simulink model "43_BusNetworkElectricityTransmissionModel"  (R2023b)
settings: Solver=VariableStepAuto  StartTime=0.0  StopTime=0.8  RelTol=1e-3
model workspace (MAT data in the model file):
  BESS_Fp_KDroop = 0.025
  BESS_KSI = 817
  BESS_PWM_fs = 560
  BESS_P_Ki = 0.5
  BESS_P_Kp = 0.0636
  BESS_Pnom = 3000000
  BESS_Q_Ki = 1
  BESS_Q_Kp = 0.0257
  BESS_Vd_Ki = 850
  BESS_Vd_Kp = 0.216
  BESS_Vnom = 1000
  BESS_Vq_KDroop = 0.025
  BESS_Vq_Ki = 850
  BESS_Vq_Kp = 0.216
  Compensation_Ki = 30
  Compensation_Kp = 3
  DC_Ki = 400
  DC_Kp = 8
  F = 0.01
  Flux_min = 0.5
  Grid_Freq_PWM = 2700
  Grid_Ireg_Ki = 5
  Grid_Ireg_Kp = 0.83
  Grid_Ireg_lim = 1.1
  Grid_Modindex_Upper = 1.1
  Grid_conv_Imax = 0.8
  H = 0.685
  Idref_max = 0.9
  Iqref_Tc = 0.3
  Ki_Var = 0.05
  Ki_Vreg = 20
  Ksh = 1.1
  L_pu = 0.3
  Llr = 0.16
  Lls = 0.18
  Lm = 2.9
  LowLoad_P = 130
  Nb_wt = 6
  P_mech = 1080000
  PeakShav_P = 200
  Pitch_Ki = 0
  Pitch_Kp = 150
  Pitch_Max = 27
  Pitch_Tc = 0.01
  Pitch_rate = 10
  Q_Filt = 50
  R_pu = 0.003
  Rotor_Freq_PWM = 1620
  Rotor_Ireg_Ki = 8
  Rotor_Ireg_Kp = 0.6
  Rotor_Ireg_lim = 0.1
  Rotor_Modindex_Upper = 2
  Rr = 0.016
  Rs = 0.023
  SOCBESS : Simulink.Parameter (value not decoded)
  T_set = 0.0001
  Tp = 5e-05
  Ts = 5e-06
  Var_C_Filt = 720000
  Var_reg_max = 1.1
  Var_reg_min = 0.9
  WT_Coeff = [0.645 116 0.4 5 21 0.00912 0.08 0.035]
  WT_H = 4.32
  WT_IGBTRon = 5.931
  WT_Param = [91.204 10143]
  Wind_Freq_Filt = 10000
  Wind_Freq_nom = 60
  Wind_P_nom = 1200000
  Wind_Rotor_V_nom = 1950
  Wind_V_nom = 500
  Zeta_Filt = 0.707106781187
  init = [-0.2 0 0 0 0 0 0 0]
  p = 3
  torque0 = 0.83
  v_Ki = 0.1
  v_Kp = 3.6
  v_Max = 1.2
  v_Min = 0.7
  v_T = 5
  vreg_max = 1
  wind_VDC_nom = 1150
  wt0 = 1.2
undefined symbols (not defined in the file): D1, D11, Delta, DiscIntNeverNeededParam, Iabc, Ion, Lithium, P, Q, Vabc
libraries: powerlib_extras x156, spsSeriesRLCBranchLib x66, spsLoadFlowBusLib x43, spsThreePhaseSeriesRLCLoadLib x33, spsThreePhaseTransformerTwoWindingsLib x32, spsThreePhaseVIMeasurementLib x30, simulink_extras x30, spsDistributedParametersLineLib x22, spsGenericPowerSystemStabilizerLib x20, spsSynchronousMachinepuStandardLib x10, spsExcitationSystemLib x10, spsHydraulicTurbineandGovernorLib x10
(part 6 of 19)

== system 43_BusNetworkElectricityTransmissionModel/ 41.4 MW Wind Generation/41.4 MW Wind Farm ==
  10.35 MW Wind Turbine 1 : Subsystem
  10.35 MW Wind Turbine 2 : Subsystem
  10.35 MW Wind Turbine 3 : Subsystem
  10.35 MW Wind Turbine 4 : Subsystem
  11.5 MVA 20KV :500V Transformer {1..4} (4 alike) : spsThreePhaseTransformerTwoWindingsLib/Three-Phase Transformer (Two Windings)  Winding1Connection=Delta (D1)  Winding2Connection=Yn  CoreType=Three single-phase transformers  SetSaturation=off  Hysteresis=off  DataFile='hysteresis'  SetInitialFlux=off  Measurements=None  UNITS=pu  NominalPower=[ 1.15e7 , 60 ]  Winding1=[ 20e3 , 0.002 , 0.08 ]  Winding2=[ 500 , 0.002 , 0.08 ]  Rm=500  Lm=500  L0=0.5  Saturation=[ 0,0 ; 0.0024,1.2 ; 1.0,1.52 ]  InitialFluxes=[ 0.8 , -0.8 , 0.7 ]  BreakLoop=off  DiscreteSolver=Trapezoidal iterative  DataType=off  TransfoNumber=1
  Control System : Subsystem
  Ground{,1..3} (4 alike) : spsGroundLib/Ground  LConnTagsString=a
  Load Flow Bus1 : spsLoadFlowBusLib/Load Flow Bus  LConnTagsString=a  Phases=single  Connectors=on one side  ID=BUS_31  Vbase=20e3  Vref=1  Vangle=0  VLF=1  VLFb=1  VLFc=1  angleLF=0  angleLFb=0  angleLFc=0
  Load Flow Bus2 : spsLoadFlowBusLib/Load Flow Bus  LConnTagsString=a  Phases=single  Connectors=on one side  ID=BUS_32  Vbase=20e3  Vref=1  Vangle=0  VLF=1  VLFb=1  VLFc=1  angleLF=0  angleLFb=0  angleLFc=0
  Load Flow Bus3 : spsLoadFlowBusLib/Load Flow Bus  LConnTagsString=a  Phases=single  Connectors=on one side  ID=BUS_33  Vbase=20e3  Vref=1  Vangle=0  VLF=1  VLFb=1  VLFc=1  angleLF=0  angleLFb=0  angleLFc=0
  Load Flow Bus4 : spsLoadFlowBusLib/Load Flow Bus  LConnTagsString=a  Phases=single  Connectors=on one side  ID=BUS_34  Vbase=500  Vref=1  Vangle=0  VLF=1  VLFb=1  VLFc=1  angleLF=0  angleLFb=0  angleLFc=0
  Load Flow Bus5 : spsLoadFlowBusLib/Load Flow Bus  LConnTagsString=a  Phases=single  Connectors=on one side  ID=BUS_35  Vbase=500  Vref=1  Vangle=0  VLF=1  VLFb=1  VLFc=1  angleLF=0  angleLFb=0  angleLFc=0
  Load Flow Bus6 : spsLoadFlowBusLib/Load Flow Bus  LConnTagsString=a  Phases=single  Connectors=on one side  ID=BUS_30  Vbase=20e3  Vref=1  Vangle=0  VLF=1  VLFb=1  VLFc=1  angleLF=0  angleLFb=0  angleLFc=0
  Load Flow Bus7 : spsLoadFlowBusLib/Load Flow Bus  LConnTagsString=a  Phases=single  Connectors=on one side  ID=BUS_36  Vbase=500  Vref=1  Vangle=0  VLF=1  VLFb=1  VLFc=1  angleLF=0  angleLFb=0  angleLFc=0
  Load Flow Bus8 : spsLoadFlowBusLib/Load Flow Bus  LConnTagsString=a  Phases=single  Connectors=on one side  ID=BUS_37  Vbase=500  Vref=1  Vangle=0  VLF=1  VLFb=1  VLFc=1  angleLF=0  angleLFb=0  angleLFc=0
  Series RLC Branch{,1..3} (4 alike) : spsSeriesRLCBranchLib/Series RLC Branch  LConnTagsString=__new0  RConnTagsString=__new0  BranchType=R  Resistance=66  Inductance=0  SetiL0=off  InitialCurrent=0  Capacitance=0  Setx0=off  InitialVoltage=0  Measurements=None
  Three-Phase PI Section Line{,1..3} (4 alike) : spsThreePhasePISectionLineLib/Three-Phase PI Section Line  LConnTagsString=a|b|c  RConnTagsString=A|B|C  Length=0.5  Frequency=60  Resistances=[ 0.01273 0.3864]  Inductances="[ 0.9337e-3  4.1264e-3]"  Capacitances=[12.74e-9 7.751e-9]
  Three-Phase Series RLC Load{,1..3} (4 alike) : spsThreePhaseSeriesRLCLoadLib/Three-Phase Series RLC Load  LConnTagsString=A|B|C  Configuration=Y (grounded)  NominalVoltage=500  Vabc=[1e3 1e3 1e3]  Vabcp=[1e3 1e3 1e3]  NominalFrequency=60  UnbalancedPower=off  ActivePower=43200  InductivePower=0  CapacitivePower=2160e3  Pabc=[10e3 9e3 11e3]  QLabc=[100 90 110]  QCabc=[100 90 110]  Pabcp=[10e3 9e3 11e3]  QLabcp=[100 90 110]  QCabcp=[100 90 110]  Measurements=None  LoadType=constant Z
  Three-Phase V-I Measurement1 : spsThreePhaseVIMeasurementLib/Three-Phase V-I Measurement  VoltageMeasurement=phase-to-ground  SetLabelV=on  LabelV=Vabc_WT2  Vpu=on  VpuLL=off  CurrentMeasurement=no  SetLabelI=on  LabelI=Iabc_WT2  Ipu=on  Pbase=2*1.8/0.9  Vbase=500  OutputType=Complex  PhasorSimulation=off  PSBequivalent=0
  Three-Phase V-I Measurement2 : spsThreePhaseVIMeasurementLib/Three-Phase V-I Measurement  VoltageMeasurement=phase-to-ground  SetLabelV=on  LabelV=Vabc_WT1  Vpu=on  VpuLL=off  CurrentMeasurement=no  SetLabelI=on  LabelI=Iabc_WT1  Ipu=off  Pbase=2*1.8/0.9  Vbase=500  OutputType=Complex  PhasorSimulation=off  PSBequivalent=0
  Three-Phase V-I Measurement3 : spsThreePhaseVIMeasurementLib/Three-Phase V-I Measurement  VoltageMeasurement=phase-to-ground  SetLabelV=on  LabelV=Vabc_WT4  Vpu=on  VpuLL=off  CurrentMeasurement=no  SetLabelI=on  LabelI=Iabc_WT4  Ipu=on  Pbase=2*1.8/0.9  Vbase=500  OutputType=Complex  PhasorSimulation=off  PSBequivalent=0
  Three-Phase V-I Measurement4 : spsThreePhaseVIMeasurementLib/Three-Phase V-I Measurement  VoltageMeasurement=phase-to-ground  SetLabelV=on  LabelV=Vabc_WT3  Vpu=on  VpuLL=off  CurrentMeasurement=no  SetLabelI=on  LabelI=Iabc_WT3  Ipu=on  Pbase=2*1.8/0.9  Vbase=500  OutputType=Complex  PhasorSimulation=off  PSBequivalent=0
  Unit Delay1 : UnitDelay  SampleTime=Ts  HasFrameUpgradeWarning=on
  A : PMIOPort  Side=Left
  B : PMIOPort  Port=2  Side=Left
  C : PMIOPort  Port=3  Side=Left
  connections:
  Three-Phase PI Section Line/RConn1 -- 11.5 MVA 20KV :500V Transformer 1/LConn1
  11.5 MVA 20KV :500V Transformer 1/LConn2 -- Three-Phase PI Section Line/RConn2
  Three-Phase PI Section Line/RConn3 -- 11.5 MVA 20KV :500V Transformer 1/LConn3
  Ground/LConn1 -- Series RLC Branch/RConn1
  Series RLC Branch/LConn1 -- 11.5 MVA 20KV :500V Transformer 1/RConn4
  11.5 MVA 20KV :500V Transformer 2/RConn1 -- Three-Phase V-I Measurement1/LConn1
  11.5 MVA 20KV :500V Transformer 2/RConn3 -- Three-Phase V-I Measurement1/LConn3
  11.5 MVA 20KV :500V Transformer 2/RConn2 -- Three-Phase V-I Measurement1/LConn2
  11.5 MVA 20KV :500V Transformer 2/RConn4 -- Series RLC Branch1/LConn1
  11.5 MVA 20KV :500V Transformer 2/LConn2 -- Three-Phase PI Section Line1/RConn2
  11.5 MVA 20KV :500V Transformer 2/LConn1 -- Three-Phase PI Section Line1/RConn1
  11.5 MVA 20KV :500V Transformer 2/LConn3 -- Three-Phase PI Section Line1/RConn3
  Ground1/LConn1 -- Series RLC Branch1/RConn1
  11.5 MVA 20KV :500V Transformer 3/RConn1 -- Three-Phase V-I Measurement4/LConn1
  11.5 MVA 20KV :500V Transformer 3/RConn3 -- Three-Phase V-I Measurement4/LConn3
  11.5 MVA 20KV :500V Transformer 3/RConn2 -- Three-Phase V-I Measurement4/LConn2
  11.5 MVA 20KV :500V Transformer 3/RConn4 -- Series RLC Branch2/LConn1
  11.5 MVA 20KV :500V Transformer 3/LConn2 -- Three-Phase PI Section Line2/RConn2
  11.5 MVA 20KV :500V Transformer 3/LConn1 -- Three-Phase PI Section Line2/RConn1
  11.5 MVA 20KV :500V Transformer 3/LConn3 -- Three-Phase PI Section Line2/RConn3
  Ground2/LConn1 -- Series RLC Branch2/RConn1
  11.5 MVA 20KV :500V Transformer 4/RConn1 -- Three-Phase V-I Measurement3/LConn1
  11.5 MVA 20KV :500V Transformer 4/RConn3 -- Three-Phase V-I Measurement3/LConn3
  11.5 MVA 20KV :500V Transformer 4/RConn2 -- Three-Phase V-I Measurement3/LConn2
  11.5 MVA 20KV :500V Transformer 4/RConn4 -- Series RLC Branch3/LConn1
  11.5 MVA 20KV :500V Transformer 4/LConn2 -- Three-Phase PI Section Line3/RConn2
  11.5 MVA 20KV :500V Transformer 4/LConn1 -- Three-Phase PI Section Line3/RConn1
  11.5 MVA 20KV :500V Transformer 4/LConn3 -- Three-Phase PI Section Line3/RConn3
  Ground3/LConn1 -- Series RLC Branch3/RConn1
  Three-Phase PI Section Line1/LConn1 -- Load Flow Bus1/LConn1 -- Three-Phase PI Section Line/LConn1 -- Load Flow Bus6/LConn1 -- Load Flow Bus3/LConn1 -- Three-Phase PI Section Line3/LConn1 -- Three-Phase PI Section Line2/LConn1 -- Load Flow Bus2/LConn1 -- A/RConn1
  Three-Phase PI Section Line1/LConn2 -- B/RConn1 -- Three-Phase PI Section Line3/LConn2 -- Three-Phase PI Section Line2/LConn2 -- Three-Phase PI Section Line/LConn2
  Three-Phase PI Section Line1/LConn3 -- C/RConn1 -- Three-Phase PI Section Line3/LConn3 -- Three-Phase PI Section Line2/LConn3 -- Three-Phase PI Section Line/LConn3
  10.35 MW Wind Turbine 2/LConn3 -- Three-Phase V-I Measurement1/RConn3 -- Three-Phase Series RLC Load1/LConn3
  10.35 MW Wind Turbine 2/LConn2 -- Three-Phase V-I Measurement1/RConn2 -- Three-Phase Series RLC Load1/LConn2
  10.35 MW Wind Turbine 2/LConn1 -- Three-Phase Series RLC Load1/LConn1 -- Load Flow Bus5/LConn1 -- Three-Phase V-I Measurement1/RConn1
  Three-Phase V-I Measurement4/RConn3 -- 10.35 MW Wind Turbine 3/LConn3 -- Three-Phase Series RLC Load2/LConn3
  Three-Phase V-I Measurement4/RConn2 -- 10.35 MW Wind Turbine 3/LConn2 -- Three-Phase Series RLC Load2/LConn2
  10.35 MW Wind Turbine 3/LConn1 -- Three-Phase Series RLC Load2/LConn1 -- Load Flow Bus7/LConn1 -- Three-Phase V-I Measurement4/RConn1
  10.35 MW Wind Turbine 4/LConn3 -- Three-Phase V-I Measurement3/RConn3 -- Three-Phase Series RLC Load3/LConn3
  10.35 MW Wind Turbine 4/LConn2 -- Three-Phase V-I Measurement3/RConn2 -- Three-Phase Series RLC Load3/LConn2
  10.35 MW Wind Turbine 4/LConn1 -- Load Flow Bus8/LConn1 -- Three-Phase V-I Measurement3/RConn1 -- Three-Phase Series RLC Load3/LConn1
  Three-Phase V-I Measurement2/LConn1 -- 11.5 MVA 20KV :500V Transformer 1/RConn1
  Three-Phase V-I Measurement2/LConn2 -- 11.5 MVA 20KV :500V Transformer 1/RConn2
  Three-Phase V-I Measurement2/LConn3 -- 11.5 MVA 20KV :500V Transformer 1/RConn3
  Three-Phase V-I Measurement2/RConn1 -- Load Flow Bus4/LConn1 -- 10.35 MW Wind Turbine 1/LConn1 -- Three-Phase Series RLC Load/LConn1
  Three-Phase V-I Measurement2/RConn2 -- 10.35 MW Wind Turbine 1/LConn2 -- Three-Phase Series RLC Load/LConn2
  Three-Phase V-I Measurement2/RConn3 -- 10.35 MW Wind Turbine 1/LConn3 -- Three-Phase Series RLC Load/LConn3

== system 43_BusNetworkElectricityTransmissionModel/400 kV Solar Farm/DC//DC Boost Converter ==
  m : Inport
  Bus Selector : BusSelector  OutputSignals=Temperature (deg C),V_PV,I_diode,Irradiance (W/m2),I_PV
  Diode : spsDiodeLib/Diode  Ron=0.0001  Lon=0  Vf=0.8  IC=0  UseSnubber=0  Rs=500  Cs=250e-9  Measurements=on
  IGBT/Diode : spsIGBTDiodeLib/IGBT//Diode  Ron=1e-3  Rs=1e5  Cs=inf  Measurements=on
  MPPT : Subsystem  mask{fp=5000, MPPT_time=2e-4, Di=0.62}
      mask prompts: fp "PWM Frequency"; MPPT_time "Time duration for MPPT"; Di "Initialization for Duty Cycle"
  Pmean Calculation : Subsystem
  Product : Product
  Series RLC Branch : spsSeriesRLCBranchLib/Series RLC Branch  LConnTagsString=__new0  RConnTagsString=__new0  BranchType=C  Resistance=1  Inductance=1e-3  SetiL0=off  InitialCurrent=0  Capacitance=1e-4  Setx0=off  InitialVoltage=0  Measurements=None
  Series RLC Branch6 : spsSeriesRLCBranchLib/Series RLC Branch  LConnTagsString=__new0  RConnTagsString=__new0  BranchType=RL  Resistance=0.005  Inductance=5e-3  SetiL0=off  InitialCurrent=0  Capacitance=0  Setx0=off  InitialVoltage=0  Measurements=None
  Step : Step  Time=0.02  SampleTime=0
  V+ : PMIOPort  Side=Left
  V- : PMIOPort  Port=2  Side=Left
  Out+ : PMIOPort  Port=3  Side=Right
  Out- : PMIOPort  Port=4  Side=Right
  tag scope: I_PV1=global, Irrad_PV1=global, Temp_PV1=global, V_PV1=global
  wires:
  [I_PV1] -> MPPT/1(PV_Current)
  Bus Selector/3 -> [I_diode]  "<I_diode>"
  m/1 -> Bus Selector/1
  Bus Selector/5 -> [I_PV1]  "<I_PV>"
  Bus Selector/1 -> [Temp_PV1]  "<Temperature (deg C)>"
  Bus Selector/2 -> [V_PV1]  "<V_PV>"
  [V_PV1] -> MPPT/2(PV_Voltage)
  Step/1 -> Product/1
  MPPT/1(Pulses) -> Product/2
  Product/1 -> IGBT/Diode/1
  Bus Selector/4 -> [Irrad_PV1]  "<Irradiance (W/m2)>"
  connections:
  Series RLC Branch/LConn1 -- V+/RConn1 -- Series RLC Branch6/LConn1
  IGBT/Diode/LConn1 -- Diode/LConn1 -- Series RLC Branch6/RConn1
  IGBT/Diode/RConn1 -- Out-/RConn1 -- V-/RConn1 -- Series RLC Branch/RConn1
  Out+/RConn1 -- Diode/RConn1

== system 43_BusNetworkElectricityTransmissionModel/400 kV Solar Farm/DC//DC Boost Converter1 ==
  m : Inport
  Bus Selector : BusSelector  OutputSignals=Temperature (deg C),V_PV,I_diode,Irradiance (W/m2),I_PV
  Deblock Converter : Step  Time=0.02  SampleTime=0
  Diode : spsDiodeLib/Diode  Ron=0.0001  Lon=0  Vf=0.8  IC=0  UseSnubber=0  Rs=inf  Cs=inf  Measurements=on
  IGBT/Diode : spsIGBTDiodeLib/IGBT//Diode  Ron=1e-3  Rs=1e5  Cs=inf  Measurements=on
  MPPT : Subsystem  mask{fp=5000, MPPT_time=2e-4, Di=0.62}
      mask prompts: fp "PWM Frequency"; MPPT_time "Time duration for MPPT"; Di "Initialization for Duty Cycle"
  Pmean Calculation : Subsystem
  Product : Product
  Series RLC Branch : spsSeriesRLCBranchLib/Series RLC Branch  LConnTagsString=__new0  RConnTagsString=__new0  BranchType=C  Resistance=1  Inductance=1e-3  SetiL0=off  InitialCurrent=0  Capacitance=1e-4  Setx0=off  InitialVoltage=0  Measurements=None
  Series RLC Branch6 : spsSeriesRLCBranchLib/Series RLC Branch  LConnTagsString=__new0  RConnTagsString=__new0  BranchType=RL  Resistance=0.005  Inductance=5e-3  SetiL0=off  InitialCurrent=0  Capacitance=0  Setx0=off  InitialVoltage=0  Measurements=None
  V+ : PMIOPort  Side=Left
  V- : PMIOPort  Port=2  Side=Left
  Out+ : PMIOPort  Port=3  Side=Right
  Out- : PMIOPort  Port=4  Side=Right
  tag scope: I_PV2=global, Irrad_PV2=global, Temp_PV2=global, V_PV2=global
  wires:
  [I_PV2] -> MPPT/1(PV_Current)
  Bus Selector/3 -> [I_diode]  "<I_diode>"
  m/1 -> Bus Selector/1
  Bus Selector/5 -> [I_PV2]  "<I_PV>"
  Bus Selector/1 -> [Temp_PV2]  "<Temperature (deg C)>"
  Bus Selector/2 -> [V_PV2]  "<V_PV>"
  Bus Selector/4 -> [Irrad_PV2]  "<Irradiance (W/m2)>"
  [V_PV2] -> MPPT/2(PV_Voltage)
  MPPT/1(Pulses) -> Product/1
  Deblock Converter/1 -> Product/2
  Product/1 -> IGBT/Diode/1
  connections:
  Series RLC Branch6/LConn1 -- Series RLC Branch/LConn1 -- V+/RConn1
  IGBT/Diode/LConn1 -- Diode/LConn1 -- Series RLC Branch6/RConn1
  V-/RConn1 -- Series RLC Branch/RConn1 -- IGBT/Diode/RConn1 -- Out-/RConn1
  Out+/RConn1 -- Diode/RConn1

== system 43_BusNetworkElectricityTransmissionModel/400 kV Solar Farm/DC//DC Boost Converter2 ==
  m : Inport
  Bus Selector : BusSelector  OutputSignals=Temperature (deg C),V_PV,I_diode,Irradiance (W/m2),I_PV
  Diode : spsDiodeLib/Diode  Ron=0.0001  Lon=0  Vf=0.8  IC=0  UseSnubber=0  Rs=inf  Cs=inf  Measurements=on
  IGBT/Diode : spsIGBTDiodeLib/IGBT//Diode  Ron=1e-3  Rs=1e5  Cs=inf  Measurements=on
  MPPT : Subsystem  mask{fp=5000, MPPT_time=2e-4, Di=0.62}
      mask prompts: fp "PWM Frequency"; MPPT_time "Time duration for MPPT"; Di "Initialization for Duty Cycle"
  Pmean Calculation : Subsystem
  Product : Product
  Series RLC Branch : spsSeriesRLCBranchLib/Series RLC Branch  LConnTagsString=__new0  RConnTagsString=__new0  BranchType=C  Resistance=1  Inductance=1e-3  SetiL0=off  InitialCurrent=0  Capacitance=1e-4  Setx0=off  InitialVoltage=0  Measurements=None
  Series RLC Branch6 : spsSeriesRLCBranchLib/Series RLC Branch  LConnTagsString=__new0  RConnTagsString=__new0  BranchType=RL  Resistance=0.005  Inductance=5e-3  SetiL0=off  InitialCurrent=0  Capacitance=0  Setx0=off  InitialVoltage=0  Measurements=None
  Step : Step  Time=0.02  SampleTime=0
  V+ : PMIOPort  Side=Left
  V- : PMIOPort  Port=2  Side=Left
  Out+ : PMIOPort  Port=3  Side=Right
  Out- : PMIOPort  Port=4  Side=Right
  tag scope: I_PV3=global, Irrad_PV3=global, Temp_PV3=global, V_PV3=global
  wires:
  [I_PV3] -> MPPT/1(PV_Current)
  Bus Selector/3 -> [I_diode]  "<I_diode>"
  m/1 -> Bus Selector/1
  Bus Selector/5 -> [I_PV3]  "<I_PV>"
  Bus Selector/1 -> [Temp_PV3]  "<Temperature (deg C)>"
  Bus Selector/2 -> [V_PV3]  "<V_PV>"
  Bus Selector/4 -> [Irrad_PV3]  "<Irradiance (W/m2)>"
  [V_PV3] -> MPPT/2(PV_Voltage)
  Step/1 -> Product/2
  MPPT/1(Pulses) -> Product/1
  Product/1 -> IGBT/Diode/1
  connections:
  Series RLC Branch6/LConn1 -- Series RLC Branch/LConn1 -- V+/RConn1
  IGBT/Diode/LConn1 -- Diode/LConn1 -- Series RLC Branch6/RConn1
  V-/RConn1 -- Series RLC Branch/RConn1 -- IGBT/Diode/RConn1 -- Out-/RConn1
  Out+/RConn1 -- Diode/RConn1

== system 43_BusNetworkElectricityTransmissionModel/400 kV Solar Farm/DC//DC Boost Converter3 ==
  m : Inport
  Bus Selector : BusSelector  OutputSignals=Temperature (deg C),V_PV,I_diode,Irradiance (W/m2),I_PV
  Diode : spsDiodeLib/Diode  Ron=0.0001  Lon=0  Vf=0.8  IC=0  UseSnubber=0  Rs=inf  Cs=inf  Measurements=on
  IGBT/Diode : spsIGBTDiodeLib/IGBT//Diode  Ron=1e-3  Rs=1e5  Cs=inf  Measurements=on
  MPPT : Subsystem  mask{fp=5000, MPPT_time=2e-4, Di=0.62}
      mask prompts: fp "PWM Frequency"; MPPT_time "Time duration for MPPT"; Di "Initialization for Duty Cycle"
  Pmean Calculation : Subsystem
  Product : Product
  Series RLC Branch : spsSeriesRLCBranchLib/Series RLC Branch  LConnTagsString=__new0  RConnTagsString=__new0  BranchType=C  Resistance=1  Inductance=1e-3  SetiL0=off  InitialCurrent=0  Capacitance=1e-4  Setx0=off  InitialVoltage=0  Measurements=None
  Series RLC Branch6 : spsSeriesRLCBranchLib/Series RLC Branch  LConnTagsString=__new0  RConnTagsString=__new0  BranchType=RL  Resistance=0.005  Inductance=5e-3  SetiL0=off  InitialCurrent=0  Capacitance=0  Setx0=off  InitialVoltage=0  Measurements=None
  Step : Step  Time=0.02  SampleTime=0
  V+ : PMIOPort  Side=Left
  V- : PMIOPort  Port=2  Side=Left
  Out+ : PMIOPort  Port=3  Side=Right
  Out- : PMIOPort  Port=4  Side=Right
  tag scope: I_PV4=global, Irrad_PV4=global, Temp_PV4=global, V_PV4=global
  wires:
  [I_PV4] -> MPPT/1(PV_Current)
  Bus Selector/3 -> [I_diode]  "<I_diode>"
  m/1 -> Bus Selector/1
  Bus Selector/5 -> [I_PV4]  "<I_PV>"
  Bus Selector/1 -> [Temp_PV4]  "<Temperature (deg C)>"
  Bus Selector/2 -> [V_PV4]  "<V_PV>"
  [V_PV4] -> MPPT/2(PV_Voltage)
  Step/1 -> Product/2
  MPPT/1(Pulses) -> Product/1
  Product/1 -> IGBT/Diode/1
  Bus Selector/4 -> [Irrad_PV4]  "<Irradiance (W/m2)>"
  connections:
  Series RLC Branch6/LConn1 -- Series RLC Branch/LConn1 -- V+/RConn1
  IGBT/Diode/LConn1 -- Diode/LConn1 -- Series RLC Branch6/RConn1
  V-/RConn1 -- Series RLC Branch/RConn1 -- IGBT/Diode/RConn1 -- Out-/RConn1
  Out+/RConn1 -- Diode/RConn1

== system 43_BusNetworkElectricityTransmissionModel/400 kV Solar Farm/VSC Control ==
  Vabc_prim : Inport  PortDimensions=3
  Iabc_prim : Inport  Port=2  PortDimensions=3
  Vdc_mes : Inport  Port=3  PortDimensions=1
  Current Regulator : Subsystem
  Iq_ref : Constant  Value=0
  Mux : Mux  Inputs=2
  PLL & Measurements : Subsystem
  PWM Generator (3-Level) : spsPWMGenerator3LevelLib/PWM Generator (3-Level)  ModulatorType=Three-phase bridge (12 pulses)  ModulatorMode=Unsynchronized  nF=27  Fc=33*60  ModulatingSignals=off  m=0.8  Freq=60  Phase=0  Ts=5e-5
  Uabc_ref Generation max (m) = 1 : Subsystem
  Unit Delay : UnitDelay  SampleTime=T_set  HasFrameUpgradeWarning=on
  VDC Regulator : Subsystem
  Vdc_ref1 : Constant  Value=Vdc_ref
  Pulses : Outport  VectorParamsAs1DForOutWhenUnconnected=off
  wires:
  VDC Regulator/1(Id_ref) -> Mux/1
  PLL & Measurements/1(wt) -> Uabc_ref Generation max (m) = 1/1(wt)
  Current Regulator/1(VdVq_conv) -> Uabc_ref Generation max (m) = 1/2(VdVq_conv)
  Iq_ref/1 -> Mux/2
  Mux/1 -> Current Regulator/3(IdIq_ref)
  PLL & Measurements/3(IdIq_prim) -> Current Regulator/2(IdIq_mes)
  PLL & Measurements/2(VdVq_prim) -> Current Regulator/1(VdVq_mes)
  Vdc_mes/1 -> VDC Regulator/1(Vdc_mes)
  Vabc_prim/1 -> PLL & Measurements/1(Vabc_prim)
  Iabc_prim/1 -> PLL & Measurements/2(Iabc_prim)
  Unit Delay/1 -> PWM Generator (3-Level)/1
  PWM Generator (3-Level)/1 -> Pulses/1
  Uabc_ref Generation max (m) = 1/1(Uabc_ref) -> Unit Delay/1
  Vdc_ref1/1 -> VDC Regulator/2(Vdc_ref)

== system 43_BusNetworkElectricityTransmissionModel/Home Network Load （with circuit breaker)/Circuit Breaker ==
  "Reset " : Inport
  Abs : Abs  SaturateOnIntegerOverflow=off
  Current Measurement1 : spsCurrentMeasurementLib/Current Measurement  PhasorSimulation=off  OutputType=Complex  PSBequivalent=0
  Data Type Conversion : DataTypeConversion  OutDataTypeStr=boolean  SaturateOnIntegerOverflow=off  RndMeth=Floor
  Data Type Conversion1 : DataTypeConversion  OutDataTypeStr=double  SaturateOnIntegerOverflow=off  RndMeth=Floor
  Hit Crossing : HitCross
  Ideal Switch : spsIdealSwitchLib/Ideal Switch  Ron=0.01  Lon=0  IC=0  Rs=1e5  Cs=inf  Measurements=on
  Logical Operator : Logic  AllPortsSameDT=off  OutDataTypeStr=boolean
  Relational Operator : RelationalOperator  Operator=<=  OutDataTypeStr=boolean  RndMeth=Simplest  InputSameDT=off
  S-R Flip-Flop : simulink_extras/Flip Flops/S-R Flip-Flop  initial_condition=0
  S-R Flip-Flop1 : simulink_extras/Flip Flops/S-R Flip-Flop  initial_condition=0
  Static Trip Current : Constant  Value=110
  Terminator : Terminator
  Terminator1 : Terminator
  Terminator2 : Terminator
  Transfer Fcn : TransferFcn  Denominator=[0.001 1]
  Connection Port1 : PMIOPort  Side=Left
  Connection Port : PMIOPort  Port=2  Side=Right
  wires:
  Logical Operator/1 -> S-R Flip-Flop1/2
  Current Measurement1/1 -> Hit Crossing/1, Abs/1
  Hit Crossing/1 -> Logical Operator/2
  Transfer Fcn/1 -> Relational Operator/1
  S-R Flip-Flop1/2 -> Terminator1/1
  Ideal Switch/1 -> Terminator2/1
  S-R Flip-Flop/1 -> Logical Operator/1
  Abs/1 -> Transfer Fcn/1
  "Reset "/1 -> Data Type Conversion/1
  S-R Flip-Flop1/1 -> Data Type Conversion1/1
  Relational Operator/1 -> S-R Flip-Flop/1
  Data Type Conversion/1 -> S-R Flip-Flop/2, S-R Flip-Flop1/1
  S-R Flip-Flop/2 -> Terminator/1
  Data Type Conversion1/1 -> Ideal Switch/1
  Static Trip Current/1 -> Relational Operator/2
  connections:
  Connection Port1/RConn1 -- Ideal Switch/LConn1
  Current Measurement1/LConn1 -- Ideal Switch/RConn1
  Connection Port/RConn1 -- Current Measurement1/RConn1

== system 43_BusNetworkElectricityTransmissionModel/Li-ion BESS/BESS ==
  ControlRoom : Inport
  BESS and Controller : Subsystem
  Bus Creator : BusCreator  Inputs=2
  Grid Measurement : Subsystem
  A : PMIOPort  Side=Left
  B : PMIOPort  Port=2  Side=Left
  C : PMIOPort  Port=3  Side=Left
  BESS_Data : Outport
  wires:
  ControlRoom/1 -> BESS and Controller/1(Control)
  BESS and Controller/1(BESS_Data) -> Bus Creator/1  "BESS"
  Bus Creator/1 -> BESS_Data/1
  Grid Measurement/1(Grid) -> Bus Creator/2, BESS and Controller/2(Grid_Data)  "Grid_Data"
  connections:
  Grid Measurement/RConn2 -- BESS and Controller/LConn2
  Grid Measurement/LConn1 -- A/RConn1
  Grid Measurement/LConn2 -- B/RConn1
  Grid Measurement/RConn3 -- BESS and Controller/LConn3
  Grid Measurement/LConn3 -- C/RConn1
  Grid Measurement/RConn1 -- BESS and Controller/LConn1

== system 43_BusNetworkElectricityTransmissionModel/Li-ion BESS/Control ==
  BESS_Data : Inport
  Bus Creator : BusCreator  Inputs=5
  Constant1 : Constant  Value=5e5  SampleTime=-1
  Constant4 : Constant  Value=-2e6  SampleTime=-1
  "Monitoring and measurement " : Subsystem
  Stair Generator : eeStairGenerator/Stair Generator  LabelModeActiveChoice=Discrete  TimeInput=[0 3]  AmplitudeInput=[1 0]  SampleTime=Ts  RepeatPattern=off  OutDataTypeStr=double
      settings: LibrarySourceBlock=ee_sl_lib/General Control/Stair Generator
  Stair Generator1 : eeStairGenerator/Stair Generator  LabelModeActiveChoice=Discrete  TimeInput=[0 3]  AmplitudeInput=[1 0]  SampleTime=Ts  RepeatPattern=off  OutDataTypeStr=double
      settings: LibrarySourceBlock=ee_sl_lib/General Control/Stair Generator
  Stair Generator3 : eeStairGenerator/Stair Generator  LabelModeActiveChoice=Discrete  TimeInput=[0 3]  AmplitudeInput=[1 0]  SampleTime=Ts  RepeatPattern=off  OutDataTypeStr=double
      settings: LibrarySourceBlock=ee_sl_lib/General Control/Stair Generator
  Control : Outport
  wires:
  Constant4/1 -> Bus Creator/2  "QRef"
  Constant1/1 -> Bus Creator/1  "PRef"
  Stair Generator1/1 -> Bus Creator/4  "PeakShav_Command"
  Stair Generator/1 -> Bus Creator/3  "Command_P"
  Bus Creator/1 -> Control/1
  BESS_Data/1 -> "Monitoring and measurement "/1(BESS_Data)
  Stair Generator3/1 -> Bus Creator/5  "BESS_Char_Command"

== system 43_BusNetworkElectricityTransmissionModel/North Network/Cs BMW- MPP8 ==
  Series RLC Branch : spsSeriesRLCBranchLib/Series RLC Branch  LConnTagsString=__new0  RConnTagsString=__new0  BranchType=C  Resistance=1  Inductance=1e-3  SetiL0=off  InitialCurrent=0  Capacitance=0.00049736  Setx0=off  InitialVoltage=0  Measurements=None
  Series RLC Branch1 : spsSeriesRLCBranchLib/Series RLC Branch  LConnTagsString=__new0  RConnTagsString=__new0  BranchType=C  Resistance=1  Inductance=1e-3  SetiL0=off  InitialCurrent=0  Capacitance=0.00049736  Setx0=off  InitialVoltage=0  Measurements=None
  Series RLC Branch2 : spsSeriesRLCBranchLib/Series RLC Branch  LConnTagsString=__new0  RConnTagsString=__new0  BranchType=C  Resistance=1  Inductance=1e-3  SetiL0=off  InitialCurrent=0  Capacitance=0.00049736  Setx0=off  InitialVoltage=0  Measurements=None
  A : PMIOPort  Side=Left
  A1 : PMIOPort  Port=2  Side=Right
  B : PMIOPort  Port=3  Side=Left
  B1 : PMIOPort  Port=4  Side=Right
  C : PMIOPort  Port=5  Side=Left
  C1 : PMIOPort  Port=6  Side=Right
  connections:
  A1/RConn1 -- Series RLC Branch/RConn1
  B1/RConn1 -- Series RLC Branch1/RConn1
  A/RConn1 -- Series RLC Branch/LConn1
  C/RConn1 -- Series RLC Branch2/LConn1
  B/RConn1 -- Series RLC Branch1/LConn1
  C1/RConn1 -- Series RLC Branch2/RConn1

== system 43_BusNetworkElectricityTransmissionModel/North Network/Cs BMWN ==
  Series RLC Branch : spsSeriesRLCBranchLib/Series RLC Branch  LConnTagsString=__new0  RConnTagsString=__new0  BranchType=C  Resistance=1  Inductance=1e-3  SetiL0=off  InitialCurrent=0  Capacitance=0.00049736  Setx0=off  InitialVoltage=0  Measurements=None
  Series RLC Branch1 : spsSeriesRLCBranchLib/Series RLC Branch  LConnTagsString=__new0  RConnTagsString=__new0  BranchType=C  Resistance=1  Inductance=1e-3  SetiL0=off  InitialCurrent=0  Capacitance=0.00049736  Setx0=off  InitialVoltage=0  Measurements=None
  Series RLC Branch2 : spsSeriesRLCBranchLib/Series RLC Branch  LConnTagsString=__new0  RConnTagsString=__new0  BranchType=C  Resistance=1  Inductance=1e-3  SetiL0=off  InitialCurrent=0  Capacitance=0.00049736  Setx0=off  InitialVoltage=0  Measurements=None
  A : PMIOPort  Side=Left
  A1 : PMIOPort  Port=2  Side=Right
  B : PMIOPort  Port=3  Side=Left
  B1 : PMIOPort  Port=4  Side=Right
  C : PMIOPort  Port=5  Side=Left
  C1 : PMIOPort  Port=6  Side=Right
  connections:
  A1/RConn1 -- Series RLC Branch/RConn1
  B1/RConn1 -- Series RLC Branch1/RConn1
  A/RConn1 -- Series RLC Branch/LConn1
  C/RConn1 -- Series RLC Branch2/LConn1
  B/RConn1 -- Series RLC Branch1/LConn1
  C1/RConn1 -- Series RLC Branch2/RConn1

== system 43_BusNetworkElectricityTransmissionModel/North Network/Cs FER ==
  Series RLC Branch : spsSeriesRLCBranchLib/Series RLC Branch  LConnTagsString=__new0  RConnTagsString=__new0  BranchType=C  Resistance=1  Inductance=1e-3  SetiL0=off  InitialCurrent=0  Capacitance=0.00049736  Setx0=off  InitialVoltage=0  Measurements=None
  Series RLC Branch1 : spsSeriesRLCBranchLib/Series RLC Branch  LConnTagsString=__new0  RConnTagsString=__new0  BranchType=C  Resistance=1  Inductance=1e-3  SetiL0=off  InitialCurrent=0  Capacitance=0.00049736  Setx0=off  InitialVoltage=0  Measurements=None
  Series RLC Branch2 : spsSeriesRLCBranchLib/Series RLC Branch  LConnTagsString=__new0  RConnTagsString=__new0  BranchType=C  Resistance=1  Inductance=1e-3  SetiL0=off  InitialCurrent=0  Capacitance=0.00049736  Setx0=off  InitialVoltage=0  Measurements=None
  A : PMIOPort  Side=Left
  A1 : PMIOPort  Port=2  Side=Right
  B : PMIOPort  Port=3  Side=Left
  B1 : PMIOPort  Port=4  Side=Right
  C : PMIOPort  Port=5  Side=Left
  C1 : PMIOPort  Port=6  Side=Right
  connections:
  A1/RConn1 -- Series RLC Branch/RConn1
  B1/RConn1 -- Series RLC Branch1/RConn1
  A/RConn1 -- Series RLC Branch/LConn1
  C/RConn1 -- Series RLC Branch2/LConn1
  B/RConn1 -- Series RLC Branch1/LConn1
  C1/RConn1 -- Series RLC Branch2/RConn1

== system 43_BusNetworkElectricityTransmissionModel/North Network/Cs LTNN ==
  Series RLC Branch : spsSeriesRLCBranchLib/Series RLC Branch  LConnTagsString=__new0  RConnTagsString=__new0  BranchType=C  Resistance=1  Inductance=1e-3  SetiL0=off  InitialCurrent=0  Capacitance=0.00049736  Setx0=off  InitialVoltage=0  Measurements=None
  Series RLC Branch1 : spsSeriesRLCBranchLib/Series RLC Branch  LConnTagsString=__new0  RConnTagsString=__new0  BranchType=C  Resistance=1  Inductance=1e-3  SetiL0=off  InitialCurrent=0  Capacitance=0.00049736  Setx0=off  InitialVoltage=0  Measurements=None
  Series RLC Branch2 : spsSeriesRLCBranchLib/Series RLC Branch  LConnTagsString=__new0  RConnTagsString=__new0  BranchType=C  Resistance=1  Inductance=1e-3  SetiL0=off  InitialCurrent=0  Capacitance=0.00049736  Setx0=off  InitialVoltage=0  Measurements=None
  A : PMIOPort  Side=Left
  A1 : PMIOPort  Port=2  Side=Right
  B : PMIOPort  Port=3  Side=Left
  B1 : PMIOPort  Port=4  Side=Right
  C : PMIOPort  Port=5  Side=Left
  C1 : PMIOPort  Port=6  Side=Right
  connections:
  A1/RConn1 -- Series RLC Branch/RConn1
  B1/RConn1 -- Series RLC Branch1/RConn1
  A/RConn1 -- Series RLC Branch/LConn1
  C/RConn1 -- Series RLC Branch2/LConn1
  B/RConn1 -- Series RLC Branch1/LConn1
  C1/RConn1 -- Series RLC Branch2/RConn1

== system 43_BusNetworkElectricityTransmissionModel/North Network/Cs ORED ==
  Series RLC Branch : spsSeriesRLCBranchLib/Series RLC Branch  LConnTagsString=__new0  RConnTagsString=__new0  BranchType=C  Resistance=1  Inductance=1e-3  SetiL0=off  InitialCurrent=0  Capacitance=0.00049736  Setx0=off  InitialVoltage=0  Measurements=None
  Series RLC Branch1 : spsSeriesRLCBranchLib/Series RLC Branch  LConnTagsString=__new0  RConnTagsString=__new0  BranchType=C  Resistance=1  Inductance=1e-3  SetiL0=off  InitialCurrent=0  Capacitance=0.00049736  Setx0=off  InitialVoltage=0  Measurements=None
  Series RLC Branch2 : spsSeriesRLCBranchLib/Series RLC Branch  LConnTagsString=__new0  RConnTagsString=__new0  BranchType=C  Resistance=1  Inductance=1e-3  SetiL0=off  InitialCurrent=0  Capacitance=0.00049736  Setx0=off  InitialVoltage=0  Measurements=None
  A : PMIOPort  Side=Left
  A1 : PMIOPort  Port=2  Side=Right
  B : PMIOPort  Port=3  Side=Left
  B1 : PMIOPort  Port=4  Side=Right
  C : PMIOPort  Port=5  Side=Left
  C1 : PMIOPort  Port=6  Side=Right
  connections:
  A1/RConn1 -- Series RLC Branch/RConn1
  B1/RConn1 -- Series RLC Branch1/RConn1
  A/RConn1 -- Series RLC Branch/LConn1
  C/RConn1 -- Series RLC Branch2/LConn1
  B/RConn1 -- Series RLC Branch1/LConn1
  C1/RConn1 -- Series RLC Branch2/RConn1

== system 43_BusNetworkElectricityTransmissionModel/North Network/Regulators 7 ==
  m : Inport
  Bus Selector : BusSelector  OutputSignals="dq0 components.Stator voltage  vq (pu),dq0 components.Stator voltage  vd (pu),Mechanical.Rotor speed  wm  (pu),Output active power   Peo (pu)"
  Constant : Constant  Value=0.8148
  Constant1 : Constant
  Math Function : Math  Operator=hypot
  Turbine and Excitation Regulators : Subsystem
  Pm : Outport
  Vf : Outport  Port=2
  tag scope: Vm7=global, w7=global
  wires:
  Bus Selector/4 -> Turbine and Excitation Regulators/3(Pe 0)  "<Output active power   Peo (pu)>"
  Constant1/1 -> Turbine and Excitation Regulators/4(Vref)
  Bus Selector/3 -> [w7], Turbine and Excitation Regulators/2(w)  "<Rotor speed  wm  (pu)>"
  Turbine and Excitation Regulators/1(Pm) -> Pm/1
  m/1 -> Bus Selector/1
  Turbine and Excitation Regulators/2(Vf) -> Vf/1
  Bus Selector/1 -> Math Function/1  "<Stator voltage  vq (pu)>"
  Math Function/1 -> [Vm7], Turbine and Excitation Regulators/5(Vm)
  Bus Selector/2 -> Math Function/2  "<Stator voltage  vd (pu)>"
  Constant/1 -> Turbine and Excitation Regulators/1(pref)

== system 43_BusNetworkElectricityTransmissionModel/North Network/Regulators 8 ==
  m : Inport
  Bus Selector : BusSelector  OutputSignals="dq0 components.Stator voltage  vq (pu),dq0 components.Stator voltage  vd (pu),Mechanical.Rotor speed  wm  (pu),Output active power   Peo (pu)"
  Constant : Constant  Value=0.935
  Constant1 : Constant
  Math Function : Math  Operator=hypot
  Turbine and Excitation Regulators : Subsystem
  Pm : Outport
  Vf : Outport  Port=2
  tag scope: Vm8=global, w8=global
  wires:
  Bus Selector/4 -> Turbine and Excitation Regulators/3(Pe 0)  "<Output active power   Peo (pu)>"
  Constant1/1 -> Turbine and Excitation Regulators/4(Vref)
  Bus Selector/3 -> [w8], Turbine and Excitation Regulators/2(w)  "<Rotor speed  wm  (pu)>"
  Turbine and Excitation Regulators/1(Pm) -> Pm/1
  m/1 -> Bus Selector/1
  Turbine and Excitation Regulators/2(Vf) -> Vf/1
  Bus Selector/1 -> Math Function/1  "<Stator voltage  vq (pu)>"
  Math Function/1 -> [Vm8], Turbine and Excitation Regulators/5(Vm)
  Bus Selector/2 -> Math Function/2  "<Stator voltage  vd (pu)>"
  Constant/1 -> Turbine and Excitation Regulators/1(pref)

== system 43_BusNetworkElectricityTransmissionModel/North Network/Regulators 9 ==
  m : Inport
  Bus Selector : BusSelector  OutputSignals="dq0 components.Stator voltage  vq (pu),dq0 components.Stator voltage  vd (pu),Mechanical.Rotor speed  wm  (pu),Output active power   Peo (pu)"
  Constant : Constant  Value=0.854
  Constant1 : Constant
  Math Function : Math  Operator=hypot
  Turbine and Excitation Regulators : Subsystem
  Pm : Outport
  Vf : Outport  Port=2
  tag scope: Vm9=global, w9=global
  wires:
  Bus Selector/4 -> Turbine and Excitation Regulators/3(Pe 0)  "<Output active power   Peo (pu)>"
  Constant1/1 -> Turbine and Excitation Regulators/4(Vref)
  Bus Selector/3 -> [w9], Turbine and Excitation Regulators/2(w)  "<Rotor speed  wm  (pu)>"
  Turbine and Excitation Regulators/1(Pm) -> Pm/1
  m/1 -> Bus Selector/1
  Turbine and Excitation Regulators/2(Vf) -> Vf/1
  Bus Selector/1 -> Math Function/1  "<Stator voltage  vq (pu)>"
  Math Function/1 -> [Vm9], Turbine and Excitation Regulators/5(Vm)
  Bus Selector/2 -> Math Function/2  "<Stator voltage  vd (pu)>"
  Constant/1 -> Turbine and Excitation Regulators/1(pref)

== system 43_BusNetworkElectricityTransmissionModel/Regulators 10/Turbine and Excitation Regulators ==
  pref : Inport
  w : Inport  Port=2
  Pe 0 : Inport  Port=3
  Vref : Inport  Port=4
  Vm : Inport  Port=5
  Add : Sum  Inputs=+-
  Complex to Real-Imag : ComplexToRealImag
  Excitation System : spsExcitationSystemLib/Excitation System  tr=20e-3  reg=[ 300, 0.001 ]  exc=[ 1, 0 ]  tgr=[ 0, 0 ]  damp=[ 0.001, 0.1 ]  sat=[ 0, 0 ]  lim=[ -11.5, 11.5, 0 ]  v0="[1.0  1.28]"
      settings: LibrarySourceBlock=sps_lib/Electrical Machines/Synchronous Machine Control/Excitation System
  Hydraulic Turbine and Governor : spsHydraulicTurbineandGovernorLib/Hydraulic Turbine and Governor  sm="[ 10/3  0.07 ]"  gate="[  0.01  0.97518  -0.1  0.1 ]"  reg="[  0.05  1.163  0.105  0  0.01  ]"  hyd="[  0  2.67  ]"  dref=0  po=0.7516
      settings: LibrarySourceBlock=|
      | sps_lib/Electrical Machines/Synchronous Machine Control/Hydraulic Turbine
      | and Governor
  Stabilitator : Subsystem
  Terminator : Terminator
  wref : Constant
  wref1 : Constant
  Pm : Outport
  Vf : Outport  Port=2
  wires:
  pref/1 -> Hydraulic Turbine and Governor/2
  Complex to Real-Imag/2 -> Excitation System/3
  wref/1 -> Hydraulic Turbine and Governor/1
  Add/1 -> Stabilitator/3(dw), Hydraulic Turbine and Governor/5
  Vm/1 -> Complex to Real-Imag/1
  Pe 0/1 -> Stabilitator/2(Pe), Hydraulic Turbine and Governor/4
  Hydraulic Turbine and Governor/2 -> Terminator/1
  Stabilitator/1(Out1) -> Excitation System/4
  w/1 -> Add/1, Hydraulic Turbine and Governor/3
  Excitation System/1 -> Vf/1
  Hydraulic Turbine and Governor/1 -> Pm/1, Stabilitator/1(Pm)
  Vref/1 -> Excitation System/1
  wref1/1 -> Add/2
  Complex to Real-Imag/1 -> Excitation System/2

== system 43_BusNetworkElectricityTransmissionModel/South Network/Cs AND ==
  Series RLC Branch : spsSeriesRLCBranchLib/Series RLC Branch  LConnTagsString=__new0  RConnTagsString=__new0  BranchType=C  Resistance=1  Inductance=1e-3  SetiL0=off  InitialCurrent=0  Capacitance=0.00049736  Setx0=off  InitialVoltage=0  Measurements=None
  Series RLC Branch1 : spsSeriesRLCBranchLib/Series RLC Branch  LConnTagsString=__new0  RConnTagsString=__new0  BranchType=C  Resistance=1  Inductance=1e-3  SetiL0=off  InitialCurrent=0  Capacitance=0.00049736  Setx0=off  InitialVoltage=0  Measurements=None
  Series RLC Branch2 : spsSeriesRLCBranchLib/Series RLC Branch  LConnTagsString=__new0  RConnTagsString=__new0  BranchType=C  Resistance=1  Inductance=1e-3  SetiL0=off  InitialCurrent=0  Capacitance=0.00049736  Setx0=off  InitialVoltage=0  Measurements=None
  A : PMIOPort  Side=Left
  A1 : PMIOPort  Port=2  Side=Right
  B : PMIOPort  Port=3  Side=Left
  B1 : PMIOPort  Port=4  Side=Right
  C : PMIOPort  Port=5  Side=Left
  C1 : PMIOPort  Port=6  Side=Right
  connections:
  A1/RConn1 -- Series RLC Branch/RConn1
  B1/RConn1 -- Series RLC Branch1/RConn1
  A/RConn1 -- Series RLC Branch/LConn1
  C/RConn1 -- Series RLC Branch2/LConn1
  B/RConn1 -- Series RLC Branch1/LConn1
  C1/RConn1 -- Series RLC Branch2/RConn1

== system 43_BusNetworkElectricityTransmissionModel/South Network/Cs CLPN ==
  Series RLC Branch : spsSeriesRLCBranchLib/Series RLC Branch  LConnTagsString=__new0  RConnTagsString=__new0  BranchType=C  Resistance=1  Inductance=1e-3  SetiL0=off  InitialCurrent=0  Capacitance=0.00049736  Setx0=off  InitialVoltage=0  Measurements=None
  Series RLC Branch1 : spsSeriesRLCBranchLib/Series RLC Branch  LConnTagsString=__new0  RConnTagsString=__new0  BranchType=C  Resistance=1  Inductance=1e-3  SetiL0=off  InitialCurrent=0  Capacitance=0.00049736  Setx0=off  InitialVoltage=0  Measurements=None
  Series RLC Branch2 : spsSeriesRLCBranchLib/Series RLC Branch  LConnTagsString=__new0  RConnTagsString=__new0  BranchType=C  Resistance=1  Inductance=1e-3  SetiL0=off  InitialCurrent=0  Capacitance=0.00049736  Setx0=off  InitialVoltage=0  Measurements=None
  A : PMIOPort  Side=Left
  A1 : PMIOPort  Port=2  Side=Right
  B : PMIOPort  Port=3  Side=Left
  B1 : PMIOPort  Port=4  Side=Right
  C : PMIOPort  Port=5  Side=Left
  C1 : PMIOPort  Port=6  Side=Right
  connections:
  A1/RConn1 -- Series RLC Branch/RConn1
  B1/RConn1 -- Series RLC Branch1/RConn1
  A/RConn1 -- Series RLC Branch/LConn1
  C/RConn1 -- Series RLC Branch2/LConn1
  B/RConn1 -- Series RLC Branch1/LConn1
  C1/RConn1 -- Series RLC Branch2/RConn1

== system 43_BusNetworkElectricityTransmissionModel/South Network/Cs CLPS ==
  Series RLC Branch : spsSeriesRLCBranchLib/Series RLC Branch  LConnTagsString=__new0  RConnTagsString=__new0  BranchType=C  Resistance=1  Inductance=1e-3  SetiL0=off  InitialCurrent=0  Capacitance=0.00049736  Setx0=off  InitialVoltage=0  Measurements=None
  Series RLC Branch1 : spsSeriesRLCBranchLib/Series RLC Branch  LConnTagsString=__new0  RConnTagsString=__new0  BranchType=C  Resistance=1  Inductance=1e-3  SetiL0=off  InitialCurrent=0  Capacitance=0.00049736  Setx0=off  InitialVoltage=0  Measurements=None
  Series RLC Branch2 : spsSeriesRLCBranchLib/Series RLC Branch  LConnTagsString=__new0  RConnTagsString=__new0  BranchType=C  Resistance=1  Inductance=1e-3  SetiL0=off  InitialCurrent=0  Capacitance=0.00049736  Setx0=off  InitialVoltage=0  Measurements=None
  A : PMIOPort  Side=Left
  A1 : PMIOPort  Port=2  Side=Right
  B : PMIOPort  Port=3  Side=Left
  B1 : PMIOPort  Port=4  Side=Right
  C : PMIOPort  Port=5  Side=Left
  C1 : PMIOPort  Port=6  Side=Right
  connections:
  A1/RConn1 -- Series RLC Branch/RConn1
  B1/RConn1 -- Series RLC Branch1/RConn1
  A/RConn1 -- Series RLC Branch/LConn1
  C/RConn1 -- Series RLC Branch2/LConn1
  B/RConn1 -- Series RLC Branch1/LConn1
  C1/RConn1 -- Series RLC Branch2/RConn1

== system 43_BusNetworkElectricityTransmissionModel/South Network/Cs CSGN ==
  Series RLC Branch : spsSeriesRLCBranchLib/Series RLC Branch  LConnTagsString=__new0  RConnTagsString=__new0  BranchType=C  Resistance=1  Inductance=1e-3  SetiL0=off  InitialCurrent=0  Capacitance=0.00049736  Setx0=off  InitialVoltage=0  Measurements=None
  Series RLC Branch1 : spsSeriesRLCBranchLib/Series RLC Branch  LConnTagsString=__new0  RConnTagsString=__new0  BranchType=C  Resistance=1  Inductance=1e-3  SetiL0=off  InitialCurrent=0  Capacitance=0.00049736  Setx0=off  InitialVoltage=0  Measurements=None
  Series RLC Branch2 : spsSeriesRLCBranchLib/Series RLC Branch  LConnTagsString=__new0  RConnTagsString=__new0  BranchType=C  Resistance=1  Inductance=1e-3  SetiL0=off  InitialCurrent=0  Capacitance=0.00049736  Setx0=off  InitialVoltage=0  Measurements=None
  A : PMIOPort  Side=Left
  A1 : PMIOPort  Port=2  Side=Right
  B : PMIOPort  Port=3  Side=Left
  B1 : PMIOPort  Port=4  Side=Right
  C : PMIOPort  Port=5  Side=Left
  C1 : PMIOPort  Port=6  Side=Right
  connections:
  A1/RConn1 -- Series RLC Branch/RConn1
  B1/RConn1 -- Series RLC Branch1/RConn1
  A/RConn1 -- Series RLC Branch/LConn1
  C/RConn1 -- Series RLC Branch2/LConn1
  B/RConn1 -- Series RLC Branch1/LConn1
  C1/RConn1 -- Series RLC Branch2/RConn1

== system 43_BusNetworkElectricityTransmissionModel/South Network/Cs MPP1D ==
  Series RLC Branch : spsSeriesRLCBranchLib/Series RLC Branch  LConnTagsString=__new0  RConnTagsString=__new0  BranchType=C  Resistance=1  Inductance=1e-3  SetiL0=off  InitialCurrent=0  Capacitance=0.00049736  Setx0=off  InitialVoltage=0  Measurements=None
  Series RLC Branch1 : spsSeriesRLCBranchLib/Series RLC Branch  LConnTagsString=__new0  RConnTagsString=__new0  BranchType=C  Resistance=1  Inductance=1e-3  SetiL0=off  InitialCurrent=0  Capacitance=0.00049736  Setx0=off  InitialVoltage=0  Measurements=None
  Series RLC Branch2 : spsSeriesRLCBranchLib/Series RLC Branch  LConnTagsString=__new0  RConnTagsString=__new0  BranchType=C  Resistance=1  Inductance=1e-3  SetiL0=off  InitialCurrent=0  Capacitance=0.00049736  Setx0=off  InitialVoltage=0  Measurements=None
  A : PMIOPort  Side=Left
  A1 : PMIOPort  Port=2  Side=Right
  B : PMIOPort  Port=3  Side=Left
  B1 : PMIOPort  Port=4  Side=Right
  C : PMIOPort  Port=5  Side=Left
  C1 : PMIOPort  Port=6  Side=Right
  connections:
  A1/RConn1 -- Series RLC Branch/RConn1
  B1/RConn1 -- Series RLC Branch1/RConn1
  A/RConn1 -- Series RLC Branch/LConn1
  C/RConn1 -- Series RLC Branch2/LConn1
  B/RConn1 -- Series RLC Branch1/LConn1
  C1/RConn1 -- Series RLC Branch2/RConn1

== system 43_BusNetworkElectricityTransmissionModel/South Network/Cs PNSM ==
  Series RLC Branch : spsSeriesRLCBranchLib/Series RLC Branch  LConnTagsString=__new0  RConnTagsString=__new0  BranchType=C  Resistance=1  Inductance=1e-3  SetiL0=off  InitialCurrent=0  Capacitance=0.00049736  Setx0=off  InitialVoltage=0  Measurements=None
  Series RLC Branch1 : spsSeriesRLCBranchLib/Series RLC Branch  LConnTagsString=__new0  RConnTagsString=__new0  BranchType=C  Resistance=1  Inductance=1e-3  SetiL0=off  InitialCurrent=0  Capacitance=0.00049736  Setx0=off  InitialVoltage=0  Measurements=None
  Series RLC Branch2 : spsSeriesRLCBranchLib/Series RLC Branch  LConnTagsString=__new0  RConnTagsString=__new0  BranchType=C  Resistance=1  Inductance=1e-3  SetiL0=off  InitialCurrent=0  Capacitance=0.00049736  Setx0=off  InitialVoltage=0  Measurements=None
  A : PMIOPort  Side=Left
  A1 : PMIOPort  Port=2  Side=Right
  B : PMIOPort  Port=3  Side=Left
  B1 : PMIOPort  Port=4  Side=Right
  C : PMIOPort  Port=5  Side=Left
  C1 : PMIOPort  Port=6  Side=Right
  connections:
  A1/RConn1 -- Series RLC Branch/RConn1
  B1/RConn1 -- Series RLC Branch1/RConn1
  A/RConn1 -- Series RLC Branch/LConn1
  C/RConn1 -- Series RLC Branch2/LConn1
  B/RConn1 -- Series RLC Branch1/LConn1
  C1/RConn1 -- Series RLC Branch2/RConn1

== system 43_BusNetworkElectricityTransmissionModel/South Network/Cs PNSN ==
  Series RLC Branch : spsSeriesRLCBranchLib/Series RLC Branch  LConnTagsString=__new0  RConnTagsString=__new0  BranchType=C  Resistance=1  Inductance=1e-3  SetiL0=off  InitialCurrent=0  Capacitance=0.00049736  Setx0=off  InitialVoltage=0  Measurements=None
  Series RLC Branch1 : spsSeriesRLCBranchLib/Series RLC Branch  LConnTagsString=__new0  RConnTagsString=__new0  BranchType=C  Resistance=1  Inductance=1e-3  SetiL0=off  InitialCurrent=0  Capacitance=0.00049736  Setx0=off  InitialVoltage=0  Measurements=None
  Series RLC Branch2 : spsSeriesRLCBranchLib/Series RLC Branch  LConnTagsString=__new0  RConnTagsString=__new0  BranchType=C  Resistance=1  Inductance=1e-3  SetiL0=off  InitialCurrent=0  Capacitance=0.00049736  Setx0=off  InitialVoltage=0  Measurements=None
  A : PMIOPort  Side=Left
  A1 : PMIOPort  Port=2  Side=Right
  B : PMIOPort  Port=3  Side=Left
  B1 : PMIOPort  Port=4  Side=Right
  C : PMIOPort  Port=5  Side=Left
  C1 : PMIOPort  Port=6  Side=Right
  connections:
  A1/RConn1 -- Series RLC Branch/RConn1
  B1/RConn1 -- Series RLC Branch1/RConn1
  A/RConn1 -- Series RLC Branch/LConn1
  C/RConn1 -- Series RLC Branch2/LConn1
  B/RConn1 -- Series RLC Branch1/LConn1
  C1/RConn1 -- Series RLC Branch2/RConn1

== system 43_BusNetworkElectricityTransmissionModel/South Network/Cs SATS ==
  Series RLC Branch : spsSeriesRLCBranchLib/Series RLC Branch  LConnTagsString=__new0  RConnTagsString=__new0  BranchType=C  Resistance=1  Inductance=1e-3  SetiL0=off  InitialCurrent=0  Capacitance=0.00049736  Setx0=off  InitialVoltage=0  Measurements=None
  Series RLC Branch1 : spsSeriesRLCBranchLib/Series RLC Branch  LConnTagsString=__new0  RConnTagsString=__new0  BranchType=C  Resistance=1  Inductance=1e-3  SetiL0=off  InitialCurrent=0  Capacitance=0.00049736  Setx0=off  InitialVoltage=0  Measurements=None
  Series RLC Branch2 : spsSeriesRLCBranchLib/Series RLC Branch  LConnTagsString=__new0  RConnTagsString=__new0  BranchType=C  Resistance=1  Inductance=1e-3  SetiL0=off  InitialCurrent=0  Capacitance=0.00049736  Setx0=off  InitialVoltage=0  Measurements=None
  A : PMIOPort  Side=Left
  A1 : PMIOPort  Port=2  Side=Right
  B : PMIOPort  Port=3  Side=Left
  B1 : PMIOPort  Port=4  Side=Right
  C : PMIOPort  Port=5  Side=Left
  C1 : PMIOPort  Port=6  Side=Right
  connections:
  A1/RConn1 -- Series RLC Branch/RConn1
  B1/RConn1 -- Series RLC Branch1/RConn1
  A/RConn1 -- Series RLC Branch/LConn1
  C/RConn1 -- Series RLC Branch2/LConn1
  B/RConn1 -- Series RLC Branch1/LConn1
  C1/RConn1 -- Series RLC Branch2/RConn1

== system 43_BusNetworkElectricityTransmissionModel/South Network/Regulators 1 ==
  m : Inport
  Bus Selector : BusSelector  OutputSignals="dq0 components.Stator voltage  vq (pu),dq0 components.Stator voltage  vd (pu),Mechanical.Rotor speed  wm  (pu),Output active power   Peo (pu)"
  Constant : Constant  Value=0.811
  Constant1 : Constant
  Math Function : Math  Operator=hypot
  Turbine and Excitation Regulators : Subsystem
  Pm : Outport
  Vf : Outport  Port=2
  tag scope: Vm1=global, w1=global
  wires:
  Constant1/1 -> Turbine and Excitation Regulators/4(Vref)
  Turbine and Excitation Regulators/1(Pm) -> Pm/1
  m/1 -> Bus Selector/1
  Turbine and Excitation Regulators/2(Vf) -> Vf/1
  Math Function/1 -> [Vm1], Turbine and Excitation Regulators/5(Vm)
  Constant/1 -> Turbine and Excitation Regulators/1(pref)
  Bus Selector/1 -> Math Function/1  "<Stator voltage  vq (pu)>"
  Bus Selector/2 -> Math Function/2  "<Stator voltage  vd (pu)>"
  Bus Selector/4 -> Turbine and Excitation Regulators/3(Pe 0)  "<Output active power   Peo (pu)>"
  Bus Selector/3 -> Turbine and Excitation Regulators/2(w), [w1]  "<Rotor speed  wm  (pu)>"
